simulink model "soal1ghesmateda"  (R2019b)
settings: Solver=VariableStepAuto  StartTime=0.0  StopTime=10  RelTol=1e-3
settings Model: Creator=user  LastModifiedBy=user

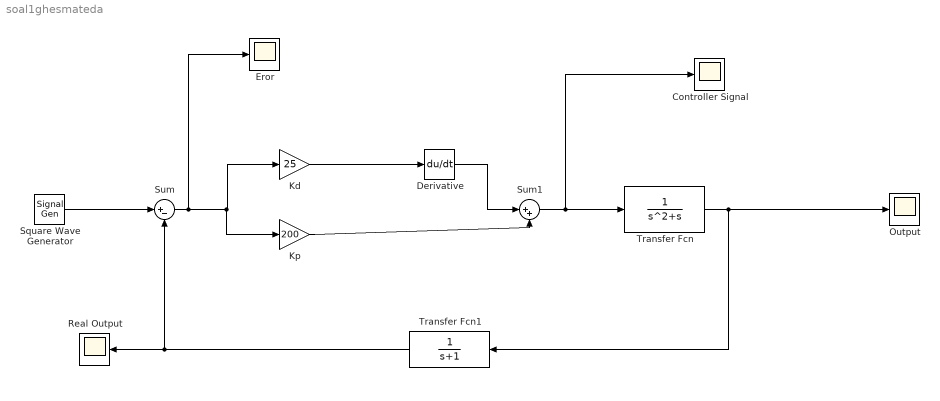
== system soal1ghesmateda ==
  Controller Signal : Scope
  Derivative : Derivative
  Eror : Scope
  "Kd " : Gain  Gain=25
  Kp : Gain  Gain=200
  "Output " : Scope
  Real Output : Scope
  "Square Wave Generator " : SignalGenerator  WaveForm=square  Amplitude=10  Frequency=2.5  Units=rad/sec
  Sum : Sum  Inputs=|+-
  Sum1 : Sum  Inputs=|++
  Transfer Fcn : TransferFcn  Denominator=[1 1 0]
  Transfer Fcn1 : TransferFcn  Denominator=[1 1]
  wires:
  "Square Wave Generator "/1 -> Sum/1
  "Kd "/1 -> Derivative/1
  Derivative/1 -> Sum1/1
  Sum1/1 -> Controller Signal/1, Transfer Fcn/1
  Kp/1 -> Sum1/2
  Sum/1 -> Eror/1, "Kd "/1, Kp/1
  Transfer Fcn/1 -> "Output "/1, Transfer Fcn1/1
  Transfer Fcn1/1 -> Real Output/1, Sum/2
